simulink model "eg_1_02_R2018a"  (R2018a)
settings: Solver=ode4  StartTime=0.0  StopTime=5  FixedStep=0.001  RelTol=1e-3  EnableMultiTasking=on
values from neighbouring files (symbols this model uses):
  k = 2    [eg_1_02b.m]    (also in eg_1_03b.m = - lqr(A,b,Q,R); eg_1_05.m; eg_1_06.m)
  kD = 3*wn*z    (= 4.2)    [eg_1_02b.m]
  kP = (3*wn^2)/2    (= 6)    [eg_1_02b.m]
  M1 = 0.5    [eg_1_02b.m]    (also in eg_1_03b.m; eg_1_05.m = 2; eg_1_06.m = 2)
  M2 = 1    [eg_1_02b.m]    (also in eg_1_03b.m; eg_1_05.m; eg_1_06.m)
  mu = 1    [eg_1_02b.m]    (also in eg_1_03b.m; eg_1_05.m = 2; eg_1_06.m = 2)
  wn = 2    [eg_1_02b.m]    (also in eg_1_02c.m = 1)
  z = 0.7    [eg_1_02b.m]
settings Model: Creator=kawata  LastModifiedBy=kawata
settings DataIOCC: LimitDataPoints=on  SaveFormat=Array  SignalLoggingSaveFormat=ModelDataLogs  SignalLoggingName=sigsOut
settings OptimizationCC: ExpressionDepthLimit=2147483647  LifeSpan=inf
settings DebuggingCC: SaveWithParameterizedLinksMsg=none  UnderspecifiedInitializationDetection=Classic  MergeDetectMultiDrivingBlocksExec=none  SignalResolutionControl=TryResolveAllWithWarning  MultiTaskDSMMsg=warning  MultiTaskCondExecSysMsg=none  FcnCallInpInsideContextMsg=warning  StateNameClashWarn=warning  SFUnexpectedBacktrackingDiag=warning  SFNoUnconditionalDefaultTransitionDiag=warning  SFExecutionAtInitializationDiag=none
settings HardwareCC: ProdBitPerPointer=32  ProdBitPerSizeT=32  ProdBitPerPtrDiffT=32  ProdLargestAtomicFloat=None  ProdIntDivRoundTo=Undefined  ProdEndianess=Unspecified  ProdWordSize=32  ProdHWDeviceType=32-bit Generic  TargetUnknown=on
settings ModelReferenceCC: PropagateSignalLabelsOutOfModel=off
settings CodeAppCC: StateflowObjectComments=on
settings GRTTargetCC: TargetLangStandard=C89/C90 (ANSI)  GeneratePreprocessorConditionals=Disable all  CombineOutputUpdateFcns=off  GRTInterface=on
settings ConfigComp: CovMetricSettings=dw  CovHtmlReporting=on  CovSaveCumulativeToWorkspaceVar=on  CovSaveSingleToWorkspaceVar=on  CovExternalEMLEnable=off

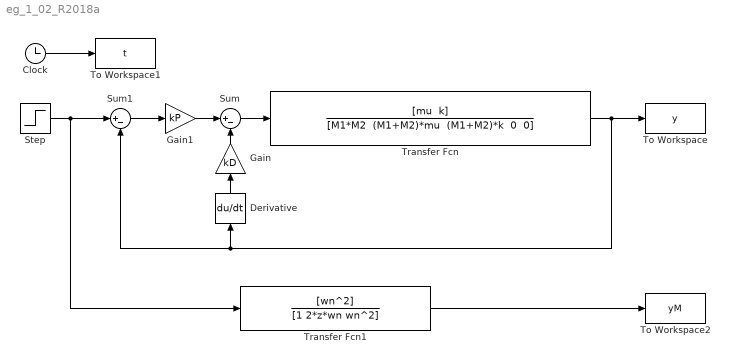
== system eg_1_02_R2018a ==
  Clock : Clock
  Derivative : Derivative
  Gain : Gain  Gain=kD  SaturateOnIntegerOverflow=on  OutDataTypeStr=Inherit: Same as input  ParamDataTypeStr=Inherit: Same as input
  Gain1 : Gain  Gain=kP  SaturateOnIntegerOverflow=on  OutDataTypeStr=Inherit: Same as input  ParamDataTypeStr=Inherit: Same as input
  Step : Step  Time=0  SampleTime=0
  Sum : Sum  Inputs=|+-  SaturateOnIntegerOverflow=on
  Sum1 : Sum  Inputs=|+-  SaturateOnIntegerOverflow=on
  To Workspace : ToWorkspace  VariableName=y  SampleTime=-1
  To Workspace1 : ToWorkspace  VariableName=t  SampleTime=-1
  To Workspace2 : ToWorkspace  VariableName=yM  SampleTime=-1
  Transfer Fcn : TransferFcn  Numerator="[mu  k]"  Denominator="[M1*M2  (M1+M2)*mu  (M1+M2)*k  0  0]"
  Transfer Fcn1 : TransferFcn  Numerator=[wn^2]  Denominator=[1 2*z*wn wn^2]
  wires:
  Transfer Fcn/1 -> Sum1/2, Derivative/1, To Workspace/1
  Derivative/1 -> Gain/1
  Sum/1 -> Transfer Fcn/1
  Sum1/1 -> Gain1/1
  Step/1 -> Sum1/1, Transfer Fcn1/1
  Clock/1 -> To Workspace1/1
  Transfer Fcn1/1 -> To Workspace2/1
  Gain1/1 -> Sum/1
  Gain/1 -> Sum/2
